simulink model "SWC_DID_type"  (R2021b)
settings: Solver=FixedStepDiscrete  StartTime=0.0  StopTime=10.0  RelTol=1e-3
settings Model: DataDictionary=APPTypes.sldd  Creator=FVT23118  LastModifiedBy=FVT23118
settings DataIOCC: SaveFormat=StructureWithTime
settings OptimizationCC: DefaultParameterBehavior=Inlined  EnhancedBackFolding=on  PassReuseOutputArgsAs=Individual arguments  ZeroExternalMemoryAtStartup=off  ZeroInternalMemoryAtStartup=off  OptimizeBlockOrder=speed  DifferentSizesBufferReuse=on  OptimizationCustomize=off  EfficientTunableParamExpr=on
settings DebuggingCC: ParameterTunabilityLossMsg=error
settings HardwareCC: ProdBitPerPointer=32  ProdBitPerSizeT=32  ProdBitPerPtrDiffT=32  ProdLargestAtomicInteger=Long  ProdLargestAtomicFloat=Double  ProdWordSize=32  ProdLongLongMode=on  ProdHWDeviceType=ARM Compatible->ARM Cortex-M
settings SFSimCC: MATLABDynamicMemAlloc=off
settings RTWCC: Description=AUTOSAR  SystemTargetFile=autosar.tlc  GenCodeOnly=on  TemplateMakefile=ert_default_tmf  PortableWordSizes=on
settings CodeAppCC: ForceParamTrailComments=on  IgnoreCustomStorageClasses=off  OperatorAnnotations=on  SimulinkDataObjDesc=on  SFDataObjDesc=on  InsertBlockDesc=on
settings STFCustomTargetCC: TargetLangStandard=C99 (ISO)  MultiwordLength=256  ParMdlRefBuildCompliant=on  CompOptLevelCompliant=on  IncludeMdlTerminateFcn=off  CombineOutputUpdateFcns=on  SuppressErrorStatus=on  ERTCustomFileBanners=on  SupportNonFinite=off  SupportComplex=off  SupportContinuousTime=off  SupportNonInlinedSFcns=off  RemoveResetFunc=on  MATLABClassNameForMDSCustomization=Simulink.SoftwareTarget.ERTCustomization  AutosarCompliant=on  GRTInterface=off  UseToolchainInfoCompliant=on  LookupTableObjectStructAxisOrder=2,1,3,4,...  LUTObjectStructOrderEvenSpacing=Size,Table,Breakpoints  SystemTargetFile=autosar.tlc
settings ERTTargetCC: TargetLangStandard=C99 (ISO)  ConcurrentExecutionCompliant=off  IncludeMdlTerminateFcn=off  SuppressErrorStatus=on  SupportNonFinite=off  SupportComplex=off  ModelStepFunctionPrototypeControlCompliant=off  CPPClassGenCompliant=off  AutosarCompliant=on  LookupTableObjectStructAxisOrder=2,1,3,4,...  LUTObjectStructOrderEvenSpacing=Size,Table,Breakpoints  GenerateASAP2=on  InlinedParameterPlacement=NonHierarchical  ERTCustomFileTemplate=example_file_process.tlc  ConvertIfToSwitch=off  SuppressUnreachableDefaultCases=off  BooleanTrueId=true_MatlabRTW  BooleanFalseId=false_MatlabRTW

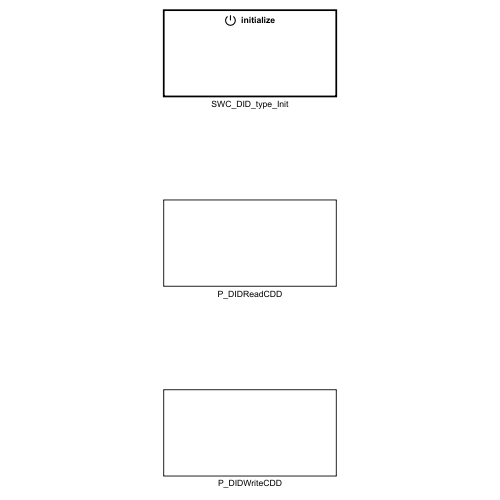
[thumbnail: Simulink's stored preview of the top-level diagram]
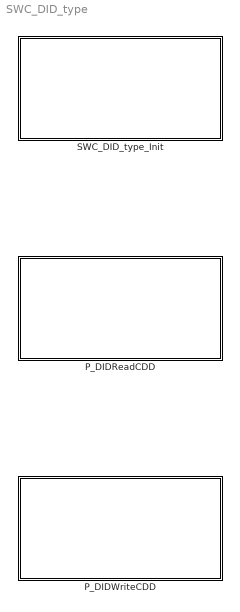
== system SWC_DID_type ==
  P_DIDReadCDD : Subsystem
  P_DIDWriteCDD : Subsystem
  SWC_DID_type_Init : Subsystem

== system SWC_DID_type/P_DIDReadCDD ==
  run_DIDGet_DKCKey_sys : Subsystem
  run_DIDGet_DynoMode_sys : Subsystem
  run_DIDGet_XWDMode_sys : Subsystem

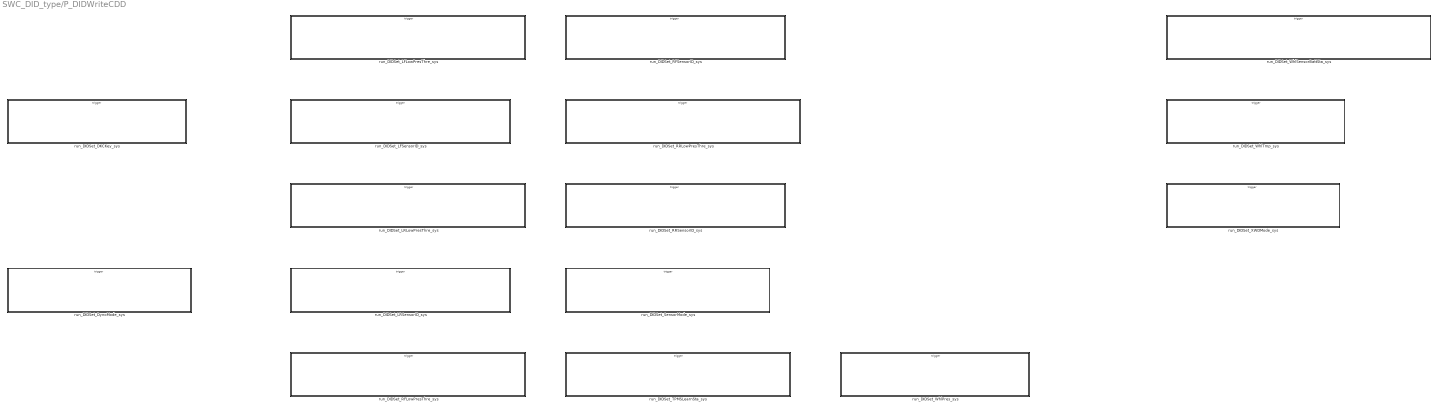
== system SWC_DID_type/P_DIDWriteCDD ==
  run_DIDSet_DKCKey_sys : Subsystem
  run_DIDSet_DynoMode_sys : Subsystem
  run_DIDSet_LFLowPresThre_sys : Subsystem
  run_DIDSet_LFSensorID_sys : Subsystem
  run_DIDSet_LRLowPresThre_sys : Subsystem
  run_DIDSet_LRSensorID_sys : Subsystem
  run_DIDSet_RFLowPresThre_sys : Subsystem
  run_DIDSet_RFSensorID_sys : Subsystem
  run_DIDSet_RRLowPresThre_sys : Subsystem
  run_DIDSet_RRSensorID_sys : Subsystem
  run_DIDSet_SensorMode_sys : Subsystem
  run_DIDSet_TPMSLearnSta_sys : Subsystem
  run_DIDSet_WhlPres_sys : Subsystem
  run_DIDSet_WhlSensorBattSta_sys : Subsystem
  run_DIDSet_WhlTmp_sys : Subsystem
  run_DIDSet_XWDMode_sys : Subsystem

== system SWC_DID_type/SWC_DID_type_Init ==
  Event Listener : EventListener  EventName=reset

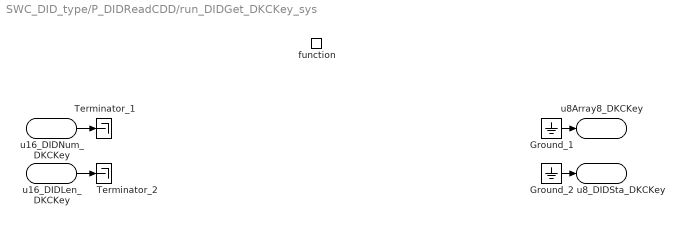
== system SWC_DID_type/P_DIDReadCDD/run_DIDGet_DKCKey_sys ==
  function : TriggerPort  TriggerType=function-call  IsSimulinkFunction=on  FunctionName=run_DIDGet_DKCKey  VariantControl=(inherit)
  Ground_1 : Ground
  Ground_2 : Ground
  Terminator_1 : Terminator
  Terminator_2 : Terminator
  u16_DIDNum_DKCKey : ArgIn  OutDataTypeStr=uint16  ArgumentName=u16_DIDNum_DKCKey
  u16_DIDLen_DKCKey : ArgIn  Port=2  OutDataTypeStr=uint16  ArgumentName=u16_DIDLen_DKCKey
  u8Array8_DKCKey : ArgOut  OutDataTypeStr=uint8  PortDimensions=8  ArgumentName=u8Array8_DKCKey
  u8_DIDSta_DKCKey : ArgOut  Port=2  OutDataTypeStr=uint8  ArgumentName=u8_DIDSta_DKCKey
  wires:
  u16_DIDNum_DKCKey/1 -> Terminator_1/1
  u16_DIDLen_DKCKey/1 -> Terminator_2/1
  Ground_1/1 -> u8Array8_DKCKey/1
  Ground_2/1 -> u8_DIDSta_DKCKey/1

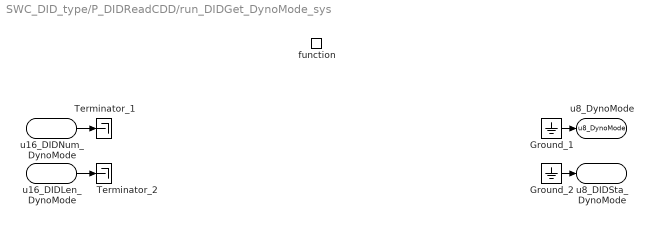
== system SWC_DID_type/P_DIDReadCDD/run_DIDGet_DynoMode_sys ==
  function : TriggerPort  TriggerType=function-call  IsSimulinkFunction=on  FunctionName=run_DIDGet_DynoMode  VariantControl=(inherit)
  Ground_1 : Ground
  Ground_2 : Ground
  Terminator_1 : Terminator
  Terminator_2 : Terminator
  u16_DIDNum_DynoMode : ArgIn  OutDataTypeStr=uint16  ArgumentName=u16_DIDNum_DynoMode
  u16_DIDLen_DynoMode : ArgIn  Port=2  OutDataTypeStr=uint16  ArgumentName=u16_DIDLen_DynoMode
  u8_DynoMode : ArgOut  OutDataTypeStr=uint8  ArgumentName=u8_DynoMode
  u8_DIDSta_DynoMode : ArgOut  Port=2  OutDataTypeStr=uint8  ArgumentName=u8_DIDSta_DynoMode
  wires:
  u16_DIDNum_DynoMode/1 -> Terminator_1/1
  u16_DIDLen_DynoMode/1 -> Terminator_2/1
  Ground_1/1 -> u8_DynoMode/1
  Ground_2/1 -> u8_DIDSta_DynoMode/1

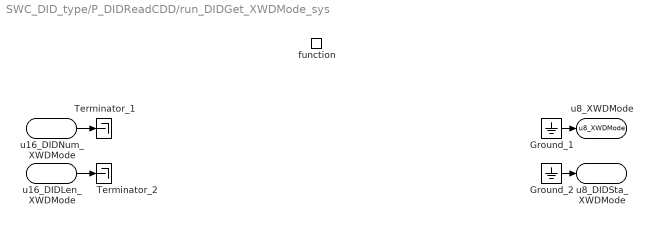
== system SWC_DID_type/P_DIDReadCDD/run_DIDGet_XWDMode_sys ==
  function : TriggerPort  TriggerType=function-call  IsSimulinkFunction=on  FunctionName=run_DIDGet_XWDMode  VariantControl=(inherit)
  Ground_1 : Ground
  Ground_2 : Ground
  Terminator_1 : Terminator
  Terminator_2 : Terminator
  u16_DIDNum_XWDMode : ArgIn  OutDataTypeStr=uint16  ArgumentName=u16_DIDNum_XWDMode
  u16_DIDLen_XWDMode : ArgIn  Port=2  OutDataTypeStr=uint16  ArgumentName=u16_DIDLen_XWDMode
  u8_XWDMode : ArgOut  OutDataTypeStr=uint8  ArgumentName=u8_XWDMode
  u8_DIDSta_XWDMode : ArgOut  Port=2  OutDataTypeStr=uint8  ArgumentName=u8_DIDSta_XWDMode
  wires:
  u16_DIDNum_XWDMode/1 -> Terminator_1/1
  u16_DIDLen_XWDMode/1 -> Terminator_2/1
  Ground_1/1 -> u8_XWDMode/1
  Ground_2/1 -> u8_DIDSta_XWDMode/1

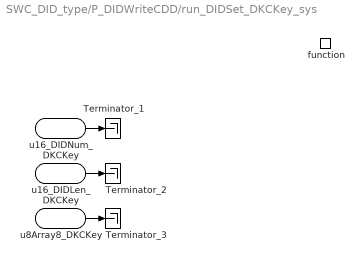
== system SWC_DID_type/P_DIDWriteCDD/run_DIDSet_DKCKey_sys ==
  function : TriggerPort  TriggerType=function-call  IsSimulinkFunction=on  FunctionName=run_DIDSet_DKCKey  VariantControl=(inherit)
  Terminator_1 : Terminator
  Terminator_2 : Terminator
  Terminator_3 : Terminator
  u16_DIDNum_DKCKey : ArgIn  OutDataTypeStr=uint16  ArgumentName=u16_DIDNum_DKCKey
  u16_DIDLen_DKCKey : ArgIn  Port=2  OutDataTypeStr=uint16  ArgumentName=u16_DIDLen_DKCKey
  u8Array8_DKCKey : ArgIn  Port=3  OutDataTypeStr=uint8  PortDimensions=8  ArgumentName=u8Array8_DKCKey
  wires:
  u16_DIDNum_DKCKey/1 -> Terminator_1/1
  u16_DIDLen_DKCKey/1 -> Terminator_2/1
  u8Array8_DKCKey/1 -> Terminator_3/1

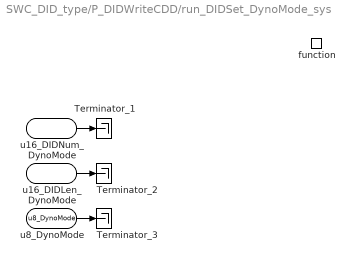
== system SWC_DID_type/P_DIDWriteCDD/run_DIDSet_DynoMode_sys ==
  function : TriggerPort  TriggerType=function-call  IsSimulinkFunction=on  FunctionName=run_DIDSet_DynoMode  VariantControl=(inherit)
  Terminator_1 : Terminator
  Terminator_2 : Terminator
  Terminator_3 : Terminator
  u16_DIDNum_DynoMode : ArgIn  OutDataTypeStr=uint16  ArgumentName=u16_DIDNum_DynoMode
  u16_DIDLen_DynoMode : ArgIn  Port=2  OutDataTypeStr=uint16  ArgumentName=u16_DIDLen_DynoMode
  u8_DynoMode : ArgIn  Port=3  OutDataTypeStr=uint8  ArgumentName=u8_DynoMode
  wires:
  u16_DIDNum_DynoMode/1 -> Terminator_1/1
  u16_DIDLen_DynoMode/1 -> Terminator_2/1
  u8_DynoMode/1 -> Terminator_3/1

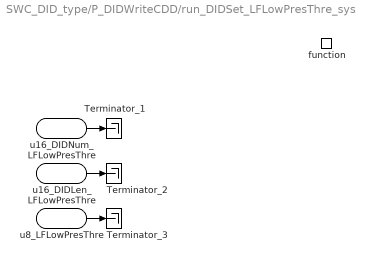
== system SWC_DID_type/P_DIDWriteCDD/run_DIDSet_LFLowPresThre_sys ==
  function : TriggerPort  TriggerType=function-call  IsSimulinkFunction=on  FunctionName=run_DIDSet_LFLowPresThre  VariantControl=(inherit)
  Terminator_1 : Terminator
  Terminator_2 : Terminator
  Terminator_3 : Terminator
  u16_DIDNum_LFLowPresThre : ArgIn  OutDataTypeStr=uint16  ArgumentName=u16_DIDNum_LFLowPresThre
  u16_DIDLen_LFLowPresThre : ArgIn  Port=2  OutDataTypeStr=uint16  ArgumentName=u16_DIDLen_LFLowPresThre
  u8_LFLowPresThre : ArgIn  Port=3  OutDataTypeStr=uint8  ArgumentName=u8_LFLowPresThre
  wires:
  u16_DIDNum_LFLowPresThre/1 -> Terminator_1/1
  u16_DIDLen_LFLowPresThre/1 -> Terminator_2/1
  u8_LFLowPresThre/1 -> Terminator_3/1

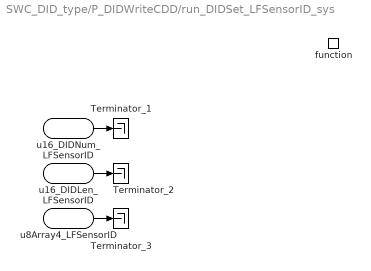
== system SWC_DID_type/P_DIDWriteCDD/run_DIDSet_LFSensorID_sys ==
  function : TriggerPort  TriggerType=function-call  IsSimulinkFunction=on  FunctionName=run_DIDSet_LFSensorID  VariantControl=(inherit)
  Terminator_1 : Terminator
  Terminator_2 : Terminator
  Terminator_3 : Terminator
  u16_DIDNum_LFSensorID : ArgIn  OutDataTypeStr=uint16  ArgumentName=u16_DIDNum_LFSensorID
  u16_DIDLen_LFSensorID : ArgIn  Port=2  OutDataTypeStr=uint16  ArgumentName=u16_DIDLen_LFSensorID
  u8Array4_LFSensorID : ArgIn  Port=3  OutDataTypeStr=uint8  PortDimensions=4  ArgumentName=u8Array4_LFSensorID
  wires:
  u16_DIDNum_LFSensorID/1 -> Terminator_1/1
  u16_DIDLen_LFSensorID/1 -> Terminator_2/1
  u8Array4_LFSensorID/1 -> Terminator_3/1

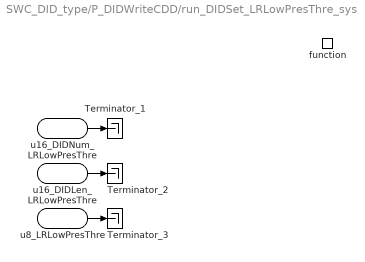
== system SWC_DID_type/P_DIDWriteCDD/run_DIDSet_LRLowPresThre_sys ==
  function : TriggerPort  TriggerType=function-call  IsSimulinkFunction=on  FunctionName=run_DIDSet_LRLowPresThre  VariantControl=(inherit)
  Terminator_1 : Terminator
  Terminator_2 : Terminator
  Terminator_3 : Terminator
  u16_DIDNum_LRLowPresThre : ArgIn  OutDataTypeStr=uint16  ArgumentName=u16_DIDNum_LRLowPresThre
  u16_DIDLen_LRLowPresThre : ArgIn  Port=2  OutDataTypeStr=uint16  ArgumentName=u16_DIDLen_LRLowPresThre
  u8_LRLowPresThre : ArgIn  Port=3  OutDataTypeStr=uint8  ArgumentName=u8_LRLowPresThre
  wires:
  u16_DIDNum_LRLowPresThre/1 -> Terminator_1/1
  u16_DIDLen_LRLowPresThre/1 -> Terminator_2/1
  u8_LRLowPresThre/1 -> Terminator_3/1

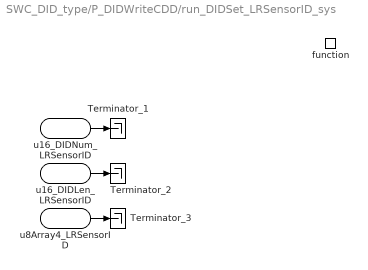
== system SWC_DID_type/P_DIDWriteCDD/run_DIDSet_LRSensorID_sys ==
  function : TriggerPort  TriggerType=function-call  IsSimulinkFunction=on  FunctionName=run_DIDSet_LRSensorID  VariantControl=(inherit)
  Terminator_1 : Terminator
  Terminator_2 : Terminator
  Terminator_3 : Terminator
  u16_DIDNum_LRSensorID : ArgIn  OutDataTypeStr=uint16  ArgumentName=u16_DIDNum_LRSensorID
  u16_DIDLen_LRSensorID : ArgIn  Port=2  OutDataTypeStr=uint16  ArgumentName=u16_DIDLen_LRSensorID
  u8Array4_LRSensorID : ArgIn  Port=3  OutDataTypeStr=uint8  PortDimensions=4  ArgumentName=u8Array4_LRSensorID
  wires:
  u16_DIDNum_LRSensorID/1 -> Terminator_1/1
  u16_DIDLen_LRSensorID/1 -> Terminator_2/1
  u8Array4_LRSensorID/1 -> Terminator_3/1

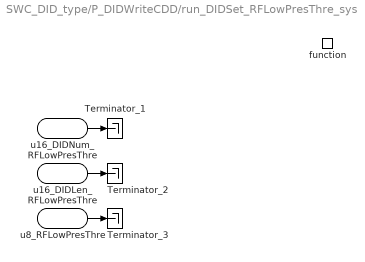
== system SWC_DID_type/P_DIDWriteCDD/run_DIDSet_RFLowPresThre_sys ==
  function : TriggerPort  TriggerType=function-call  IsSimulinkFunction=on  FunctionName=run_DIDSet_RFLowPresThre  VariantControl=(inherit)
  Terminator_1 : Terminator
  Terminator_2 : Terminator
  Terminator_3 : Terminator
  u16_DIDNum_RFLowPresThre : ArgIn  OutDataTypeStr=uint16  ArgumentName=u16_DIDNum_RFLowPresThre
  u16_DIDLen_RFLowPresThre : ArgIn  Port=2  OutDataTypeStr=uint16  ArgumentName=u16_DIDLen_RFLowPresThre
  u8_RFLowPresThre : ArgIn  Port=3  OutDataTypeStr=uint8  ArgumentName=u8_RFLowPresThre
  wires:
  u16_DIDNum_RFLowPresThre/1 -> Terminator_1/1
  u16_DIDLen_RFLowPresThre/1 -> Terminator_2/1
  u8_RFLowPresThre/1 -> Terminator_3/1

== system SWC_DID_type/P_DIDWriteCDD/run_DIDSet_RFSensorID_sys ==
  function : TriggerPort  TriggerType=function-call  IsSimulinkFunction=on  FunctionName=run_DIDSet_RFSensorID  VariantControl=(inherit)
  Terminator_1 : Terminator
  Terminator_2 : Terminator
  Terminator_3 : Terminator
  u16_DIDNum_RFSensorID : ArgIn  OutDataTypeStr=uint16  ArgumentName=u16_DIDNum_RFSensorID
  u16_DIDLen_RFSensorID : ArgIn  Port=2  OutDataTypeStr=uint16  ArgumentName=u16_DIDLen_RFSensorID
  u8Array4_RFSensorID : ArgIn  Port=3  OutDataTypeStr=uint8  PortDimensions=4  ArgumentName=u8Array4_RFSensorID
  wires:
  u16_DIDNum_RFSensorID/1 -> Terminator_1/1
  u16_DIDLen_RFSensorID/1 -> Terminator_2/1
  u8Array4_RFSensorID/1 -> Terminator_3/1

== system SWC_DID_type/P_DIDWriteCDD/run_DIDSet_RRLowPresThre_sys ==
  function : TriggerPort  TriggerType=function-call  IsSimulinkFunction=on  FunctionName=run_DIDSet_RRLowPresThre  VariantControl=(inherit)
  Terminator_1 : Terminator
  Terminator_2 : Terminator
  Terminator_3 : Terminator
  u16_DIDNum_RRLowPresThre : ArgIn  OutDataTypeStr=uint16  ArgumentName=u16_DIDNum_RRLowPresThre
  u16_DIDLen_RRLowPresThre : ArgIn  Port=2  OutDataTypeStr=uint16  ArgumentName=u16_DIDLen_RRLowPresThre
  u8_RRLowPresThre : ArgIn  Port=3  OutDataTypeStr=uint8  ArgumentName=u8_RRLowPresThre
  wires:
  u16_DIDNum_RRLowPresThre/1 -> Terminator_1/1
  u16_DIDLen_RRLowPresThre/1 -> Terminator_2/1
  u8_RRLowPresThre/1 -> Terminator_3/1

== system SWC_DID_type/P_DIDWriteCDD/run_DIDSet_RRSensorID_sys ==
  function : TriggerPort  TriggerType=function-call  IsSimulinkFunction=on  FunctionName=run_DIDSet_RRSensorID  VariantControl=(inherit)
  Terminator_1 : Terminator
  Terminator_2 : Terminator
  Terminator_3 : Terminator
  u16_DIDNum_RRSensorID : ArgIn  OutDataTypeStr=uint16  ArgumentName=u16_DIDNum_RRSensorID
  u16_DIDLen_RRSensorID : ArgIn  Port=2  OutDataTypeStr=uint16  ArgumentName=u16_DIDLen_RRSensorID
  u8Array4_RRSensorID : ArgIn  Port=3  OutDataTypeStr=uint8  PortDimensions=4  ArgumentName=u8Array4_RRSensorID
  wires:
  u16_DIDNum_RRSensorID/1 -> Terminator_1/1
  u16_DIDLen_RRSensorID/1 -> Terminator_2/1
  u8Array4_RRSensorID/1 -> Terminator_3/1

== system SWC_DID_type/P_DIDWriteCDD/run_DIDSet_SensorMode_sys ==
  function : TriggerPort  TriggerType=function-call  IsSimulinkFunction=on  FunctionName=run_DIDSet_SensorMode  VariantControl=(inherit)
  Terminator_1 : Terminator
  Terminator_2 : Terminator
  Terminator_3 : Terminator
  u16_DIDNum_SensorMode : ArgIn  OutDataTypeStr=uint16  ArgumentName=u16_DIDNum_SensorMode
  u16_DIDLen_SensorMode : ArgIn  Port=2  OutDataTypeStr=uint16  ArgumentName=u16_DIDLen_SensorMode
  u8_SensorMode : ArgIn  Port=3  OutDataTypeStr=uint8  ArgumentName=u8_SensorMode
  wires:
  u16_DIDNum_SensorMode/1 -> Terminator_1/1
  u16_DIDLen_SensorMode/1 -> Terminator_2/1
  u8_SensorMode/1 -> Terminator_3/1

== system SWC_DID_type/P_DIDWriteCDD/run_DIDSet_TPMSLearnSta_sys ==
  function : TriggerPort  TriggerType=function-call  IsSimulinkFunction=on  FunctionName=run_DIDSet_TPMSLearnSta  VariantControl=(inherit)
  Terminator_1 : Terminator
  Terminator_2 : Terminator
  Terminator_3 : Terminator
  u16_DIDNum_TPMSLearnSta : ArgIn  OutDataTypeStr=uint16  ArgumentName=u16_DIDNum_TPMSLearnSta
  u16_DIDLen_TPMSLearnSta : ArgIn  Port=2  OutDataTypeStr=uint16  ArgumentName=u16_DIDLen_TPMSLearnSta
  u8_TPMSLearnSta : ArgIn  Port=3  OutDataTypeStr=uint8  ArgumentName=u8_TPMSLearnSta
  wires:
  u16_DIDNum_TPMSLearnSta/1 -> Terminator_1/1
  u16_DIDLen_TPMSLearnSta/1 -> Terminator_2/1
  u8_TPMSLearnSta/1 -> Terminator_3/1

== system SWC_DID_type/P_DIDWriteCDD/run_DIDSet_WhlPres_sys ==
  function : TriggerPort  TriggerType=function-call  IsSimulinkFunction=on  FunctionName=run_DIDSet_WhlPres  VariantControl=(inherit)
  Terminator_1 : Terminator
  Terminator_2 : Terminator
  Terminator_3 : Terminator
  u16_DIDNum_WhlPres : ArgIn  OutDataTypeStr=uint16  ArgumentName=u16_DIDNum_WhlPres
  u16_DIDLen_WhlPres : ArgIn  Port=2  OutDataTypeStr=uint16  ArgumentName=u16_DIDLen_WhlPres
  u8Array4_WhlPres : ArgIn  Port=3  OutDataTypeStr=uint8  PortDimensions=4  ArgumentName=u8Array4_WhlPres
  wires:
  u16_DIDNum_WhlPres/1 -> Terminator_1/1
  u16_DIDLen_WhlPres/1 -> Terminator_2/1
  u8Array4_WhlPres/1 -> Terminator_3/1

== system SWC_DID_type/P_DIDWriteCDD/run_DIDSet_WhlSensorBattSta_sys ==
  function : TriggerPort  TriggerType=function-call  IsSimulinkFunction=on  FunctionName=run_DIDSet_WhlSensorBattSta  VariantControl=(inherit)
  Terminator_1 : Terminator
  Terminator_2 : Terminator
  Terminator_3 : Terminator
  u16_DIDNum_WhlSensorBattSta : ArgIn  OutDataTypeStr=uint16  ArgumentName=u16_DIDNum_WhlSensorBattSta
  u16_DIDLen_WhlSensorBattSta : ArgIn  Port=2  OutDataTypeStr=uint16  ArgumentName=u16_DIDLen_WhlSensorBattSta
  u8_WhlSensorBattSta : ArgIn  Port=3  OutDataTypeStr=uint8  ArgumentName=u8_WhlSensorBattSta
  wires:
  u16_DIDNum_WhlSensorBattSta/1 -> Terminator_1/1
  u16_DIDLen_WhlSensorBattSta/1 -> Terminator_2/1
  u8_WhlSensorBattSta/1 -> Terminator_3/1

== system SWC_DID_type/P_DIDWriteCDD/run_DIDSet_WhlTmp_sys ==
  function : TriggerPort  TriggerType=function-call  IsSimulinkFunction=on  FunctionName=run_DIDSet_WhlTmp  VariantControl=(inherit)
  Terminator_1 : Terminator
  Terminator_2 : Terminator
  Terminator_3 : Terminator
  u16_DIDNum_WhlTmp : ArgIn  OutDataTypeStr=uint16  ArgumentName=u16_DIDNum_WhlTmp
  u16_DIDLen_WhlTmp : ArgIn  Port=2  OutDataTypeStr=uint16  ArgumentName=u16_DIDLen_WhlTmp
  u8Array4_WhlTmp : ArgIn  Port=3  OutDataTypeStr=uint8  PortDimensions=4  ArgumentName=u8Array4_WhlTmp
  wires:
  u16_DIDNum_WhlTmp/1 -> Terminator_1/1
  u16_DIDLen_WhlTmp/1 -> Terminator_2/1
  u8Array4_WhlTmp/1 -> Terminator_3/1

== system SWC_DID_type/P_DIDWriteCDD/run_DIDSet_XWDMode_sys ==
  function : TriggerPort  TriggerType=function-call  IsSimulinkFunction=on  FunctionName=run_DIDSet_XWDMode  VariantControl=(inherit)
  Terminator_1 : Terminator
  Terminator_2 : Terminator
  Terminator_3 : Terminator
  u16_DIDNum_XWDMode : ArgIn  OutDataTypeStr=uint16  ArgumentName=u16_DIDNum_XWDMode
  u16_DIDLen_XWDMode : ArgIn  Port=2  OutDataTypeStr=uint16  ArgumentName=u16_DIDLen_XWDMode
  u8_XWDMode : ArgIn  Port=3  OutDataTypeStr=uint8  ArgumentName=u8_XWDMode
  wires:
  u16_DIDNum_XWDMode/1 -> Terminator_1/1
  u16_DIDLen_XWDMode/1 -> Terminator_2/1
  u8_XWDMode/1 -> Terminator_3/1
